simulink model "kalman_filter_test"  (R2021b)
settings: Solver=FixedStepAuto  StartTime=0.0  StopTime=120  FixedStep=Ts  RelTol=1e-3
InitFcn:
  | load_params;
values from neighbouring files (symbols this model uses):
  P0 = 9.9e-05    [load_params.m]
  Q = [1e-4; 1e-2; 10]    [load_params.m]
  R = 1e-4    (= 0.0001)    [load_params.m]
  Ts = 0.001    [load_params.m]
  x0 = [simin(1, 2:end)'; zeros(order-3, 1)]    [load_params.m]
libraries: simulink x4
settings Model: Creator=sgirardi  LastModifiedBy=sgirardi
settings DataIOCC: SaveOutput=off  DSMLogging=off  SaveTime=off  ReturnWorkspaceOutputs=off

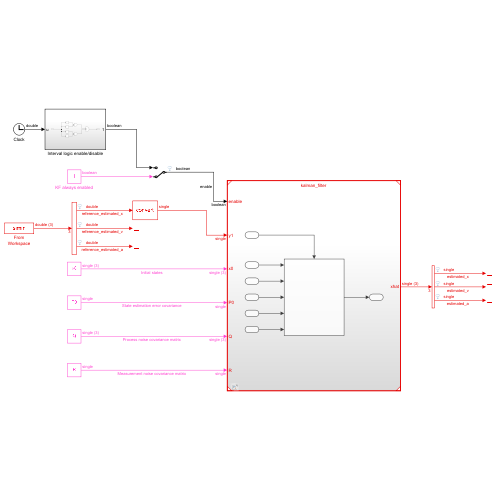
[thumbnail: Simulink's stored preview of the top-level diagram]
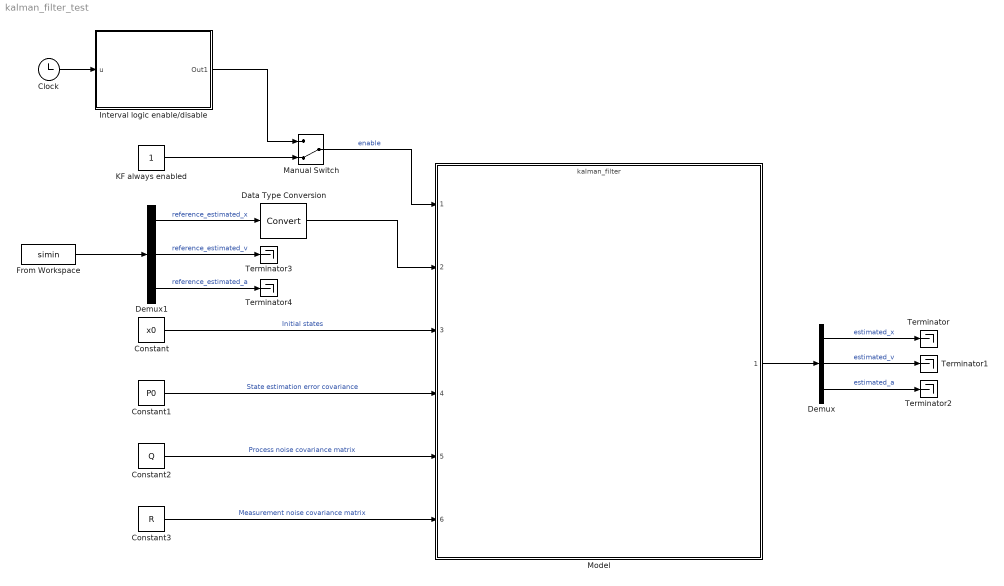
== system kalman_filter_test ==
  Clock : Clock
  Constant : Constant  Value=x0  OutDataTypeStr=single
  Constant1 : Constant  Value=P0  OutDataTypeStr=single
  Constant2 : Constant  Value=Q  OutDataTypeStr=single
  Constant3 : Constant  Value=R  OutDataTypeStr=single
  Data Type Conversion : DataTypeConversion
  Demux : Demux  Outputs=3
  Demux1 : Demux  Outputs=3
  From Workspace : FromWorkspace  VariableName=simin  SampleTime=Ts  Interpolate=off  OutputAfterFinalValue=Holding final value
  Interval logic enable/disable : Subsystem
  KF always enabled : Constant  OutDataTypeStr=boolean
  Manual Switch : ManualSwitch  CurrentSetting=0
  Model : ModelReference  ModelNameDialog=kalman_filter.slx  SimulationMode=Normal  ModelReferenceVersion=1.10
  Terminator{,1..4} (5 alike) : Terminator
  wires:
  Model/1 -> Demux/1
  Constant/1 -> Model/3  "Initial states"
  Constant1/1 -> Model/4  "State estimation error covariance"
  Constant3/1 -> Model/6  "Measurement noise covariance matrix"
  Constant2/1 -> Model/5  "Process noise covariance matrix"
  From Workspace/1 -> Demux1/1
  Demux1/1 -> Data Type Conversion/1  "reference_estimated_x"
  Data Type Conversion/1 -> Model/2
  Demux/1 -> Terminator/1  "estimated_x"
  Demux/2 -> Terminator1/1  "estimated_v"
  Demux/3 -> Terminator2/1  "estimated_a"
  Demux1/2 -> Terminator3/1  "reference_estimated_v"
  Demux1/3 -> Terminator4/1  "reference_estimated_a"
  Clock/1 -> Interval logic enable/disable/1(u)
  Interval logic enable/disable/1(Out1) -> Manual Switch/1
  Manual Switch/1 -> Model/1  "enable"
  KF always enabled/1 -> Manual Switch/2

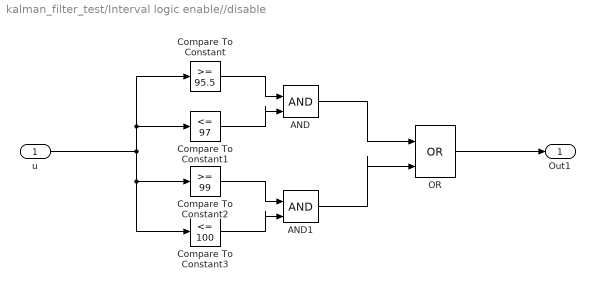
== system kalman_filter_test/Interval logic enable//disable ==
  u : Inport
  AND : Logic  IconShape=distinctive  AllPortsSameDT=off  OutDataTypeStr=boolean
  AND1 : Logic  IconShape=distinctive  AllPortsSameDT=off  OutDataTypeStr=boolean
  Compare To Constant : simulink/Logic and Bit Operations/Compare To Constant  relop=>=  const=95.5  OutDataTypeStr=boolean
  Compare To Constant1 : simulink/Logic and Bit Operations/Compare To Constant  relop=<=  const=97  OutDataTypeStr=boolean
  Compare To Constant2 : simulink/Logic and Bit Operations/Compare To Constant  relop=>=  const=99  OutDataTypeStr=boolean
  Compare To Constant3 : simulink/Logic and Bit Operations/Compare To Constant  relop=<=  const=100  OutDataTypeStr=boolean
  OR : Logic  Operator=OR  IconShape=distinctive  AllPortsSameDT=off  OutDataTypeStr=boolean
  Out1 : Outport
  wires:
  Compare To Constant3/1 -> AND1/2
  Compare To Constant1/1 -> AND/2
  AND1/1 -> OR/2
  Compare To Constant2/1 -> AND1/1
  u/1 -> Compare To Constant3/1, Compare To Constant2/1, Compare To Constant/1, Compare To Constant1/1
  AND/1 -> OR/1
  Compare To Constant/1 -> AND/1
  OR/1 -> Out1/1
